simulink model "deadbeat1sim"  (Simulink 7.1)
settings: Solver=ode1  StartTime=0.0  StopTime=20  FixedStep=0.01/f  RelTol=1e-3
values from neighbouring files (symbols this model uses):
  f = handles.f    [aliasing.m]    (also in approx.m = fvec(i); approxctrl.m = fvec(i); approxctrl2.m = fvec(i); boded.m = fvec(i))
libraries: cstblocks x3
settings Model: Creator=rpm  LastModifiedBy=rpm
settings DataIOCC: LimitDataPoints=off  SaveOutput=off  SignalLogging=off  TimeSaveName=t

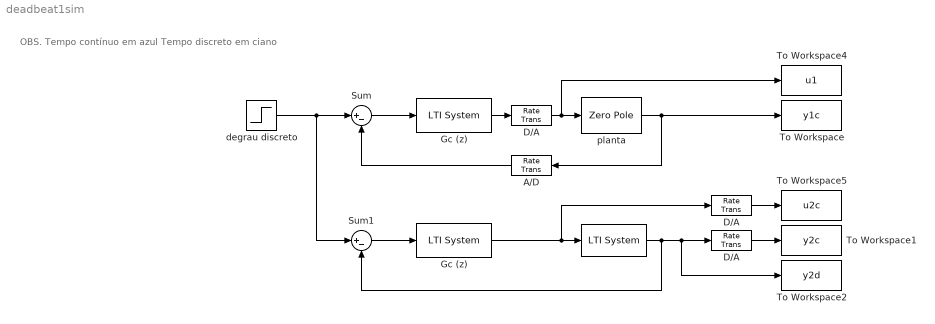
== system deadbeat1sim ==
  note: OBS.
      | Tempo contínuo em azul
      | Tempo discreto em ciano
  " " : cstblocks/LTI System  SystemSampleTime=-1  sys=Gpz  IC=[]
  "  D/A  " : RateTransition  Integrity=off  Deterministic=off  OutPortSampleTimeOpt=Inherit  OutPortSampleTime=0
  " D/A " : RateTransition  Integrity=off  Deterministic=off  OutPortSampleTimeOpt=Inherit  OutPortSampleTime=0
  " Gc (z) " : cstblocks/LTI System  SystemSampleTime=-1  sys=Gcz  IC=[]
  A/D : RateTransition  Orientation=left  OutPortSampleTime=1/f
  D/A : RateTransition  Integrity=off  Deterministic=off  OutPortSampleTimeOpt=Inherit  OutPortSampleTime=0
  Gc (z) : cstblocks/LTI System  SystemSampleTime=-1  sys=Gcz  IC=[]
  Sum : Sum  Inputs=|+-  OutDataType=sfix(16)  OutScaling=2^0  SampleTime=1/f
  Sum1 : Sum  Inputs=|+-  OutDataType=sfix(16)  OutScaling=2^0  SampleTime=1/f
  To Workspace : ToWorkspace  VariableName=y1c  SampleTime=-1  SaveFormat=Structure
  To Workspace1 : ToWorkspace  VariableName=y2c  SampleTime=-1  SaveFormat=Structure
  To Workspace2 : ToWorkspace  VariableName=y2d  SampleTime=-1  SaveFormat=Structure
  To Workspace4 : ToWorkspace  VariableName=u1  SampleTime=-1  SaveFormat=Structure
  To Workspace5 : ToWorkspace  VariableName=u2c  SampleTime=-1  SaveFormat=Structure
  degrau discreto : Step  Time=0  SampleTime=1/f
  planta : ZeroPole  Zeros=[]  Poles=[0 -0.1]  Gain=[0.1]
  wires:
  Gc (z)/1 -> D/A/1
  Sum/1 -> Gc (z)/1
  planta/1 -> To Workspace/1, A/D/1
  " Gc (z) "/1 -> " "/1, " D/A "/1
  Sum1/1 -> " Gc (z) "/1
  " "/1 -> Sum1/2, "  D/A  "/1, To Workspace2/1
  degrau discreto/1 -> Sum/1, Sum1/1
  A/D/1 -> Sum/2
  D/A/1 -> planta/1, To Workspace4/1
  " D/A "/1 -> To Workspace5/1
  "  D/A  "/1 -> To Workspace1/1
